simulink model "sys_sim"  (R2024b)
settings: Solver=VariableStepAuto  StartTime=0.0  StopTime=8  RelTol=1e-3  AbsTol=1e-3  EnableMultiTasking=on
values from neighbouring files (symbols this model uses):
  N = Nm+mp*(x2+L*(theta2*cos(theta)-theta1^2*sin(theta)))    [sys_calc.m]
undefined symbols (not defined in the file or in its folder): X, Y, Z
libraries: sm_lib x62, nesl_utility x19, slpidlib x2
(part 1 of 3)
settings Model: Creator=Skythinker  LastModifiedBy=hanze
settings SolverCC: AutoScaleAbsTol=off  ZeroCrossAlgorithm=Adaptive  AlgebraicLoopSolver=TrustRegion  MaxZcPerStep=1
settings DataIOCC: LimitDataPoints=on  MaxDataPoints=10000
settings OptimizationCC: ReuseModelBlockBuffer=off  LifeSpan=inf
settings DebuggingCC: MaskedZcDiagnostic=none  IgnoredZcDiagnostic=none  UnconnectedInputMsg=warning  UnconnectedOutputMsg=warning  UnconnectedLineMsg=warning  AllowSymbolicDim=off  SFUnexpectedBacktrackingDiag=warning  SFNoUnconditionalDefaultTransitionDiag=warning  SFExecutionAtInitializationDiag=none  ArithmeticOperatorsInVariantConditions=warning
settings ModelReferenceCC: EnableRefExpFcnMdlSchedulingChecks=on
settings SFSimCC: SimUseLocalCustomCode=off  CustomCodeUndefinedFunction=UseInterfaceOnly
settings RTWCC: RTWUseLocalCustomCode=off  GPUComputeCapability=3.5  DLArmComputeVersion=19.05
settings CodeAppCC: StateflowObjectComments=on
settings GRTTargetCC: TargetLangStandard=C89/C90 (ANSI)
settings ConfigComp: CovMetricSettings=dw  CovSaveCumulativeToWorkspaceVar=on  CovSaveSingleToWorkspaceVar=on  CovExternalEMLEnable=off  CovSFcnEnable=off
settings SimscapeCC: SimscapeLogType=all  SimscapeLogSimulationStatistics=on  SimscapeLogDataHistory=10000

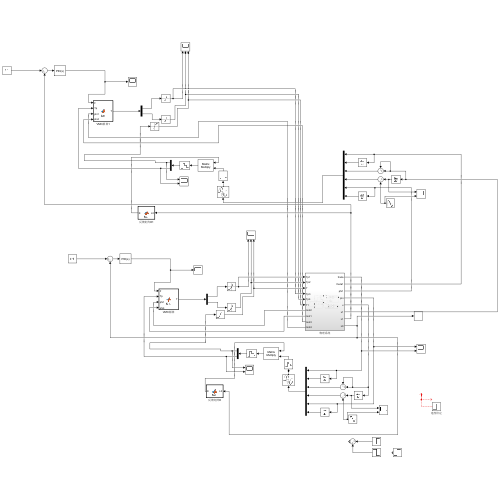
[thumbnail: Simulink's stored preview of the top-level diagram]
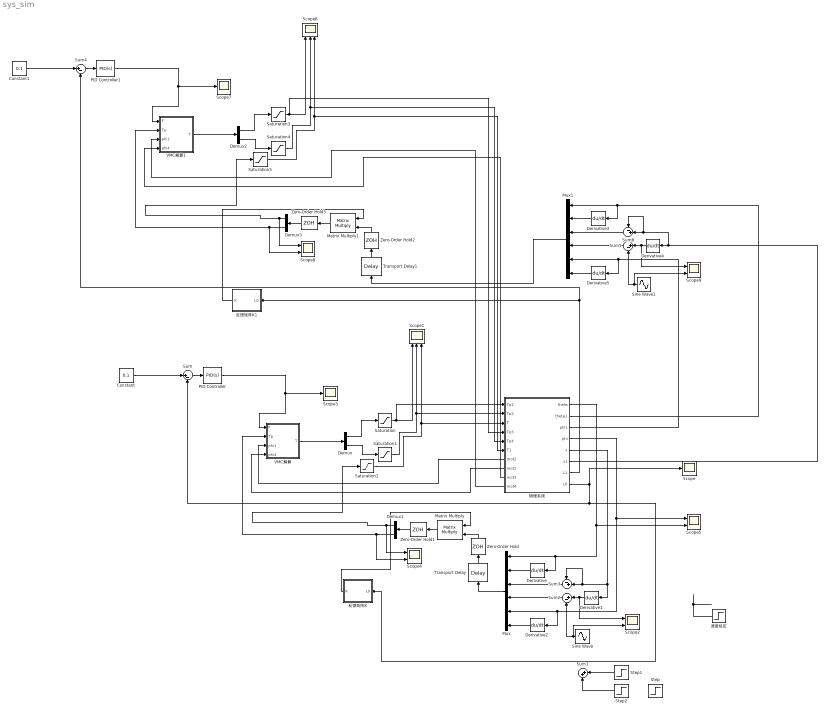
== system sys_sim ==
  Constant : Constant  Value=0.1
  Constant1 : Constant  Value=0.1
  Demux{,1..3} (4 alike) : Demux  Outputs=2
  Derivative{,1..5} (6 alike) : Derivative
  Matrix Multiply : Product  Multiplication=Matrix(*)
  Matrix Multiply1 : Product  Multiplication=Matrix(*)
  Mux : Mux  Inputs=6
  Mux1 : Mux  Inputs=6
  PID Controller : slpidlib/PID Controller  Controller=PID  Form=Parallel  TimeDomain=Continuous-time  UseExternalTs=off  SampleTime=-1  IntegratorMethod=Forward Euler  FilterMethod=Forward Euler  ControllerParametersSource=internal  P=100  I=500  UseKiTs=off  D=5  UseExternalDerivativeSource=off  N=100  UseFilter=on  TunerSelectOption=Transfer Function Based (PID Tuner App)  InitialConditionSource=internal  InitialConditionForIntegrator=0  InitialConditionForFilter=0  DifferentiatorICPrevScaledInput=0  ExternalReset=none  TrackingMode=off  Kt=1  LimitOutput=off  SatLimitsSource=internal  UpperSaturationLimit=inf  LowerSaturationLimit=-inf  LinearizeAsGain=on  AntiWindupMode=none  Kb=1  LimitIntegrator=off  UpperIntegratorSaturationLimit=1.5  LowerIntegratorSaturationLimit=-1.5  POutMin=[]  POutMax=[]  IOutMin=[]  IOutMax=[]  DOutMin=[]  DOutMax=[]  NOutMin=[]  NOutMax=[]  SumOutMin=[]  SumOutMax=[]  SaturationOutMin=[]  SaturationOutMax=[]  PParamMin=[]  PParamMax=[]  IParamMin=[]  IParamMax=[]  DParamMin=[]  DParamMax=[]  NParamMin=[]  NParamMax=[]  KbParamMin=[]  KbParamMax=[]  KtParamMin=[]  KtParamMax=[]  KbOutMin=[]  KbOutMax=[]  KtOutMin=[]  KtOutMax=[]  IntegratorOutMin=[]  IntegratorOutMax=[]  FilterOutMin=[]  FilterOutMax=[]  SumI1OutMin=[]  SumI1OutMax=[]  SumI2OutMin=[]  SumI2OutMax=[]  SumI3OutMin=[]  SumI3OutMax=[]  SumI4OutMin=[]  SumI4OutMax=[]  SumDOutMin=[]  SumDOutMax=[]  DifferentiatorOutMin=[]  DifferentiatorOutMax=[]  FilterDiffOutCoefMin=[]  FilterDiffOutCoefMax=[]  ReciprocalOutMin=[]  ReciprocalOutMax=[]  SumDenOutMin=[]  SumDenOutMax=[]  SumNumOutMin=[]  SumNumOutMax=[]  DivideOutMin=[]  DivideOutMax=[]  UdiffTsProdOutMin=[]  UdiffTsProdOutMax=[]  NTsProdOutMin=[]  NTsProdOutMax=[]  UintegralTsProdOutMin=[]  UintegralTsProdOutMax=[]  UngainTsProdOutMin=[]  UngainTsProdOutMax=[]  ClampingZeroOutDataTypeStr=Inherit: Inherit via back propagation  ClampingZeroOutMin=[]  ClampingZeroOutMax=[]  FilterDenConstantOutDataTypeStr=Inherit: Inherit via back propagation  FilterDenConstantOutMin=[]  FilterDenConstantOutMax=[]  PCopyOutDataTypeStr=Inherit: Inherit via back propagation  PCopyOutMin=[]  PCopyOutMax=[]  NCopyOutDataTypeStr=Inherit: Inherit via back propagation  NCopyOutMin=[]  NCopyOutMax=[]  IntegratorContinuousStateAttributes=''  IntegratorStateMustResolveToSignalObject=off  IntegratorRTWStateStorageClass=Auto  FilterContinuousStateAttributes=''  FilterStateMustResolveToSignalObject=off  FilterRTWStateStorageClass=Auto  ParallelPVariant=InternalParameters  IdealPVariant=Disabled  IVariant=InternalParameters  DVariant=InternalParameters  IntegratorVariant=Continuous  SatVariant=Disabled  AWVariant=Passthrough  PCopyVariant=Disabled  TRVariant=Disabled  FdbkBlocksVariant=Forward  IdealPFdbkVariant=Disabled  SatFdbkVariant=Disabled  DerivativeFilterVariant=ContFilter  NVariant=InternalParameters  NCopyVariant=Disabled  FilterICVariant=InternalICsFilter  IntegratorICVariant=InternalICs  ExternalResetVariant=Disabled  TRSumVariant=Passthrough  SumFdbkVariant=Disabled  SumVariant=Sum_PID  TsampFilterVariant=InternalTs  TsampNgainVariant=Passthrough  TsampIntegralVariant=Disabled_SignalSpec  ExternalSaturationOutDataTypeStr=Inherit: Same as second input  DerivativeSourceVariant=ErrorSignal  PreIntVariant=InternalPreInt
  PID Controller1 : slpidlib/PID Controller  Controller=PID  Form=Parallel  TimeDomain=Continuous-time  UseExternalTs=off  SampleTime=-1  IntegratorMethod=Forward Euler  FilterMethod=Forward Euler  ControllerParametersSource=internal  P=100  I=500  UseKiTs=off  D=5  UseExternalDerivativeSource=off  N=100  UseFilter=on  TunerSelectOption=Transfer Function Based (PID Tuner App)  InitialConditionSource=internal  InitialConditionForIntegrator=0  InitialConditionForFilter=0  DifferentiatorICPrevScaledInput=0  ExternalReset=none  TrackingMode=off  Kt=1  LimitOutput=off  SatLimitsSource=internal  UpperSaturationLimit=inf  LowerSaturationLimit=-inf  LinearizeAsGain=on  AntiWindupMode=none  Kb=1  LimitIntegrator=off  UpperIntegratorSaturationLimit=1.5  LowerIntegratorSaturationLimit=-1.5  POutMin=[]  POutMax=[]  IOutMin=[]  IOutMax=[]  DOutMin=[]  DOutMax=[]  NOutMin=[]  NOutMax=[]  SumOutMin=[]  SumOutMax=[]  SaturationOutMin=[]  SaturationOutMax=[]  PParamMin=[]  PParamMax=[]  IParamMin=[]  IParamMax=[]  DParamMin=[]  DParamMax=[]  NParamMin=[]  NParamMax=[]  KbParamMin=[]  KbParamMax=[]  KtParamMin=[]  KtParamMax=[]  KbOutMin=[]  KbOutMax=[]  KtOutMin=[]  KtOutMax=[]  IntegratorOutMin=[]  IntegratorOutMax=[]  FilterOutMin=[]  FilterOutMax=[]  SumI1OutMin=[]  SumI1OutMax=[]  SumI2OutMin=[]  SumI2OutMax=[]  SumI3OutMin=[]  SumI3OutMax=[]  SumI4OutMin=[]  SumI4OutMax=[]  SumDOutMin=[]  SumDOutMax=[]  DifferentiatorOutMin=[]  DifferentiatorOutMax=[]  FilterDiffOutCoefMin=[]  FilterDiffOutCoefMax=[]  ReciprocalOutMin=[]  ReciprocalOutMax=[]  SumDenOutMin=[]  SumDenOutMax=[]  SumNumOutMin=[]  SumNumOutMax=[]  DivideOutMin=[]  DivideOutMax=[]  UdiffTsProdOutMin=[]  UdiffTsProdOutMax=[]  NTsProdOutMin=[]  NTsProdOutMax=[]  UintegralTsProdOutMin=[]  UintegralTsProdOutMax=[]  UngainTsProdOutMin=[]  UngainTsProdOutMax=[]  ClampingZeroOutDataTypeStr=Inherit: Inherit via back propagation  ClampingZeroOutMin=[]  ClampingZeroOutMax=[]  FilterDenConstantOutDataTypeStr=Inherit: Inherit via back propagation  FilterDenConstantOutMin=[]  FilterDenConstantOutMax=[]  PCopyOutDataTypeStr=Inherit: Inherit via back propagation  PCopyOutMin=[]  PCopyOutMax=[]  NCopyOutDataTypeStr=Inherit: Inherit via back propagation  NCopyOutMin=[]  NCopyOutMax=[]  IntegratorContinuousStateAttributes=''  IntegratorStateMustResolveToSignalObject=off  IntegratorRTWStateStorageClass=Auto  FilterContinuousStateAttributes=''  FilterStateMustResolveToSignalObject=off  FilterRTWStateStorageClass=Auto  ParallelPVariant=InternalParameters  IdealPVariant=Disabled  IVariant=InternalParameters  DVariant=InternalParameters  IntegratorVariant=Continuous  SatVariant=Disabled  AWVariant=Passthrough  PCopyVariant=Disabled  TRVariant=Disabled  FdbkBlocksVariant=Forward  IdealPFdbkVariant=Disabled  SatFdbkVariant=Disabled  DerivativeFilterVariant=ContFilter  NVariant=InternalParameters  NCopyVariant=Disabled  FilterICVariant=InternalICsFilter  IntegratorICVariant=InternalICs  ExternalResetVariant=Disabled  TRSumVariant=Passthrough  SumFdbkVariant=Disabled  SumVariant=Sum_PID  TsampFilterVariant=InternalTs  TsampNgainVariant=Passthrough  TsampIntegralVariant=Disabled_SignalSpec  ExternalSaturationOutDataTypeStr=Inherit: Same as second input  DerivativeSourceVariant=ErrorSignal  PreIntVariant=InternalPreInt
  Saturation{,1,3..4} (4 alike) : Saturate  UpperLimit=0.15  LowerLimit=-0.15  ZeroCross=off
  Saturation2 : Saturate  UpperLimit=0.03  LowerLimit=-0.03  ZeroCross=off
  Saturation5 : Saturate  UpperLimit=0.03  LowerLimit=-0.03  ZeroCross=off
  Scope : Scope
  Scope1 : Scope  NumInputPorts=3
  Scope{2,4..5,8..9} (5 alike) : Scope  NumInputPorts=2
  Scope3 : Scope
  Scope6 : Scope  NumInputPorts=3
  Scope7 : Scope
  Sine Wave : Sin  Frequency=1.5  SampleTime=0
  Sine Wave1 : Sin  Frequency=1.5  SampleTime=0
  Step : Step  Time=0.2  After=0.3  SampleTime=0
  Step1 : Step  Time=0.2  After=0.8  SampleTime=0
  Step2 : Step  Time=4  After=-0.8  SampleTime=0
  Sum{,2,4..5} (4 alike) : Sum  Inputs=|+-
  Sum1 : Sum  Inputs=|++
  Sum3 : Sum  Inputs=-+|
  Sum6 : Sum  Inputs=-+|
  Transport Delay : TransportDelay  DelayTime=0
  Transport Delay1 : TransportDelay  DelayTime=0
  VMC解算 : MATLAB Function  TreatAsAtomicUnit=on
  VMC解算1 : MATLAB Function  TreatAsAtomicUnit=on
  Zero-Order Hold{,1..3} (4 alike) : ZeroOrderHold  SampleTime=0.005
  反馈矩阵K : MATLAB Function  TreatAsAtomicUnit=on
  反馈矩阵K1 : MATLAB Function  TreatAsAtomicUnit=on
  物理系统 : Subsystem
      settings: PortSchema="{\"entries\":[{\"content\":{\"sides\":[{\"content\":{\"connectorIds\":[\"In1\",\"In2\",\"In3\",\"In4\",\"In5\",\"In6\",\"Out9\",\"Out10\",\"Out11\",\"Out12\"]},\"type\":\"ConnectorPlacement.EquallySpacedRectSide\",\"uuid\":\"664d59a3-0a31-49e2-bbc6-fa33d49ec8c0\"},{\"content\":{\"connectorIds\":[\"Out1\",\"Out2\",\"Out3\",\"Out4\",\"Out5\",\"Out6\",\"Out7\",\"Out8\"],\"side\":\"RIGHT\"},\"type\":\"ConnectorPlacement.EquallySpacedRectSide\",\"uuid\":\"d048cd87-328e-45c8-839d-92aa139afc03\"},{\"content\":{\"side\":\"TOP\"},\"type\":\"ConnectorPlacement.EquallySpacedRectSide\",\"uuid\":\"f5424ee2-3185-467c-8de4-9f4b544a14b9\"}]},\"type\":\"ConnectorPlacement.EquallySpacedConnector\",\"uuid\":\"b3bc5ba0-ba30-4936-a275-c2533c1238aa\"}],\"packageUris\":[\"http://schema.mathworks.com/mf0/Connector/R2020b\"],\"version\":\"1.0\"}"
  速度给定 : Step  SampleTime=0
  wires:
  Demux/2 -> Saturation1/1
  Demux/1 -> Saturation/1
  VMC解算/1(T) -> Demux/1
  Saturation/1 -> 物理系统/1(Tp1), Scope1/1
  Saturation1/1 -> Scope1/2, 物理系统/2(Tp2)
  Sum/1 -> PID Controller/1
  物理系统/8(L0) -> 反馈矩阵K/1(L0), Sum/2, Scope/1
  Constant/1 -> Sum/1
  PID Controller/1 -> VMC解算/1(F), Scope3/1
  物理系统/10(mot1) -> VMC解算/4(phi4)
  物理系统/9(mot2) -> VMC解算/3(phi1)
  Matrix Multiply/1 -> Zero-Order Hold1/1
  反馈矩阵K/1(K) -> Matrix Multiply/1
  物理系统/1(theta) -> Scope5/2, Derivative/1, Mux/1
  Derivative/1 -> Mux/2
  物理系统/5(x) -> Sum3/1, Sum3/2, Derivative1/1
  Derivative1/1 -> Scope2/1, Sum2/1
  Derivative2/1 -> Mux/6
  Demux1/1 -> Saturation2/1, Scope4/1
  Saturation2/1 -> Scope1/3, 物理系统/3(T)
  Sum2/1 -> Mux/4
  Step1/1 -> Sum1/1
  Step2/1 -> Sum1/2
  物理系统/4(phi) -> Scope5/1, Mux/5, Derivative2/1
  Demux1/2 -> VMC解算/2(Tp), Scope4/2
  Zero-Order Hold/1 -> Matrix Multiply/2
  Zero-Order Hold1/1 -> Demux1/1
  Transport Delay/1 -> Zero-Order Hold/1
  Mux/1 -> Transport Delay/1
  Sum3/1 -> Mux/3
  速度给定/1 -> ?
  Sine Wave/1 -> Scope2/2, Sum2/2
  Demux3/1 -> Saturation5/1, Scope8/1
  Saturation5/1 -> 物理系统/6(T1), Scope6/3
  物理系统/11(mot3) -> VMC解算1/4(phi4)
  Saturation4/1 -> 物理系统/5(Tp4), Scope6/2
  反馈矩阵K1/1(K) -> Matrix Multiply1/1
  物理系统/12(mot4) -> VMC解算1/3(phi1)
  VMC解算1/1(T) -> Demux2/1
  Saturation3/1 -> 物理系统/4(Tp3), Scope6/1
  Transport Delay1/1 -> Zero-Order Hold2/1
  Demux3/2 -> VMC解算1/2(Tp), Scope8/2
  Mux1/1 -> Transport Delay1/1
  PID Controller1/1 -> VMC解算1/1(F), Scope7/1
  Zero-Order Hold3/1 -> Demux3/1
  Demux2/1 -> Saturation3/1
  Demux2/2 -> Saturation4/1
  物理系统/7(L1) -> Sum4/2, 反馈矩阵K1/1(L0)
  Sum4/1 -> PID Controller1/1
  Matrix Multiply1/1 -> Zero-Order Hold3/1
  Constant1/1 -> Sum4/1
  Zero-Order Hold2/1 -> Matrix Multiply1/2
  Derivative4/1 -> Scope9/1, Sum5/1
  Derivative5/1 -> Mux1/6
  Sum5/1 -> Mux1/4
  物理系统/6(x1) -> Sum6/1, Sum6/2, Derivative4/1
  Sum6/1 -> Mux1/3
  Sine Wave1/1 -> Scope9/2, Sum5/2
  物理系统/2(theta1) -> Mux1/1, Derivative3/1
  Derivative3/1 -> Mux1/2
  物理系统/3(phi1) -> Mux1/5, Derivative5/1
